simulink model "dblpend2"  (Simulink 6.0)
settings: Solver=ode45  SolverMode=SingleTasking  StartTime=0  StopTime=10000  MaxStep=0.05  RelTol=1e-5  AbsTol=1e-6
PreLoadFcn:
  | l2=58.4154;w2=14.5619;n=1.084;e=.1478;
settings Model: Creator=The MathWorks Inc.  LastModifiedBy=batserve  ExtModeAutoUpdateStatusClock=off
settings DataIOCC: ExternalInput=[]  InitialState=[]  LimitDataPoints=off  SaveOutput=off  SaveTime=off
settings OptimizationCC: BooleanDataType=off
settings DebuggingCC: CheckExecutionContextPreStartOutputMsg=on  CheckExecutionContextRuntimeOutputMsg=on  SolverPrmCheckMsg=none
settings HardwareCC: TargetUnknown=on

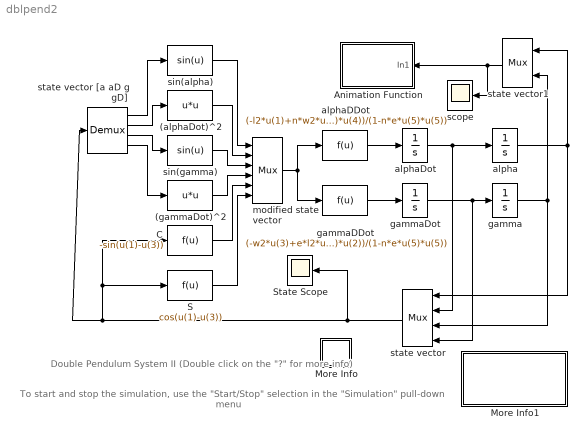
== system dblpend2 ==
  note: Double Pendulum System II
      | (Double click on the "?" for more info)
  note: To start and stop the simulation, use the "Start/Stop"
      | selection in the "Simulation" pull-down menu
  (alphaDot)^2 : Fcn  Expr=u*u
  (gammaDot)^2 : Fcn  Expr=u*u
  Animation Function : Subsystem  Orientation=left  PropExecContextAcrossSSBoundary=on
      mask Display: disp('pndanim3')
  C : Fcn  Expr=-sin(u(1)-u(3))
  More Info : Subsystem  PropExecContextAcrossSSBoundary=on
      mask Display: disp('?')
  More Info1 : Subsystem  PropExecContextAcrossSSBoundary=on
      settings: OpenFcn=simcad(bdroot)
      mask Display: disp('Double click\nhere for\nSIMULINK Help')
  S : Fcn  Expr=cos(u(1)-u(3))
  State Scope : Scope
      settings: TickLabels=on  TimeRange=40.000000  DataFormat=Array
  alpha : Integrator  InitialCondition=0*(pi/180)
  alphaDDot : Fcn  Expr=(-l2*u(1)+n*w2*u(5)*u(3)-n*e*u(5)*u(6)*u(2)-n*u(6)*u(4))/(1-n*e*u(5)*u(5))
  alphaDot : Integrator
  gamma : Integrator  InitialCondition=80*(pi/180)
  gammaDDot : Fcn  Expr=(-w2*u(3)+e*l2*u(5)*u(1)+n*e*u(5)*u(6)*u(4)+e*u(6)*u(2))/(1-n*e*u(5)*u(5))
  gammaDot : Integrator
  modified state vector : Mux  Inputs=6
  scope : Scope
      settings: TickLabels=on  TimeRange=60.000000  DataFormat=Array
  sin(alpha) : Fcn  Expr=sin(u)
  sin(gamma) : Fcn  Expr=sin(u)
  state vector : Mux  Orientation=left
  state vector [a aD g gD] : Demux
  state vector1 : Mux  Orientation=left  Inputs=2
  wires:
  alphaDDot/1 -> alphaDot/1
  gammaDDot/1 -> gammaDot/1
  alphaDot/1 -> alpha/1, state vector/2
  gammaDot/1 -> gamma/1, state vector/4
  alpha/1 -> state vector/1, state vector1/1
  gamma/1 -> state vector/3, state vector1/2
  state vector1/1 -> Animation Function/1(In1), scope/1
  state vector/1 -> state vector [a aD g gD]/1, C/1, S/1, State Scope/1
  sin(alpha)/1 -> modified state vector/1
  (alphaDot)^2/1 -> modified state vector/2
  sin(gamma)/1 -> modified state vector/3
  (gammaDot)^2/1 -> modified state vector/4
  C/1 -> modified state vector/5
  S/1 -> modified state vector/6
  modified state vector/1 -> alphaDDot/1, gammaDDot/1
  state vector [a aD g gD]/4 -> (gammaDot)^2/1
  state vector [a aD g gD]/3 -> sin(gamma)/1
  state vector [a aD g gD]/2 -> (alphaDot)^2/1
  state vector [a aD g gD]/1 -> sin(alpha)/1

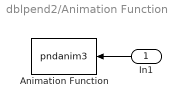
== system dblpend2/Animation Function ==
  In1 : Inport  Orientation=left  Port=1  LatchInput=off
  Animation Function : S-Function  Orientation=left  FunctionName=pndanim3  Parameters=0.05
      settings: DeleteFcn=if ~isempty(findobj('type','figure','name','dblpend2 Animation'));close('dblpend2 Animation'); end;
  wires:
  In1/1 -> Animation Function/1

== system dblpend2/More Info ==
  note: Try experimenting with different initial conditions for
      | alpha and gamma to see some remarkable behavior.
      | This system exhibits very strong nonlinear coupling.
  note: This system models a double pendulum system where
      | the rest state has the pendulums balanced to hang
      | at right angles to one another
  note: Associated with the demo is an animation function that
      | will automatically open a figure window and display to it.

== system dblpend2/More Info1 ==
  note: This system models a double pendulum system where
      | the rest state has both pendulums hanging vertically.
  note: Associated with the demo is an animation function that
      | will automatically open a figure window and display to it.
  note: Try experimenting with different initial conditions for
      | alpha and gamma to see the unusal coupling effects.
